simulink model "AOO_VOO_Mode"  (R2023b)
settings: Solver=VariableStepAuto  StartTime=0.0  StopTime=10.0  RelTol=1e-3
undefined symbols (not defined in the file): D10, D11, D12, D13, D2, D4, D5, D7, D8, D9, PTA0, PTA2, PTB23, PTB9, PTC3, PTC4, PTD0, PTD1, PTD2, PTD3
libraries: frdmk64flib x10
settings Model: Creator=haley  LastModifiedBy=haley

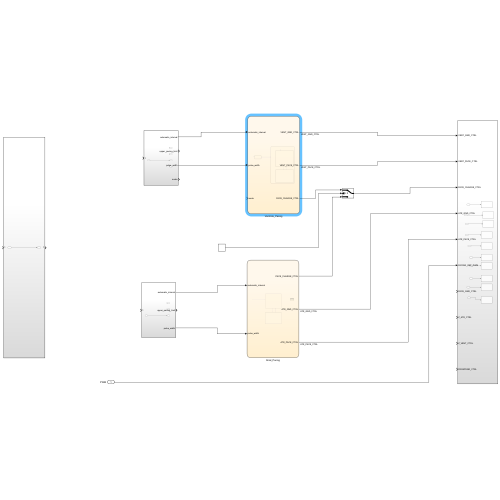
[thumbnail: Simulink's stored preview of the top-level diagram]
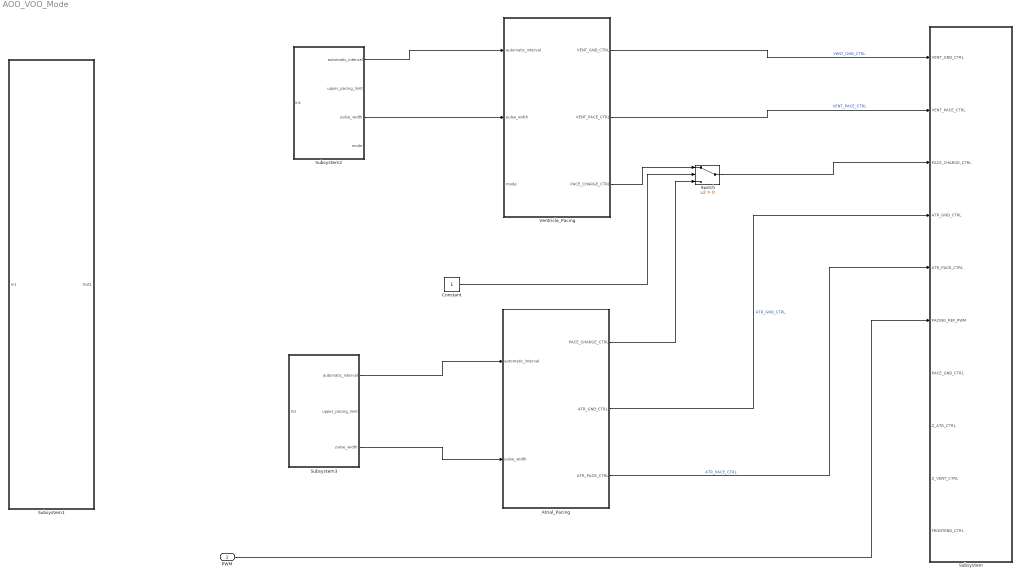
== system AOO_VOO_Mode ==
  PWM : Inport
  Atrial_Pacing : Stateflow chart  TreatAsAtomicUnit=on
      settings: PortSchema="{\"entries\":[{\"content\":{\"sides\":[{\"content\":{\"connectorIds\":[\"In1\",\"In2\"]},\"type\":\"ConnectorPlacement.EquallySpacedRectSide\",\"uuid\":\"6ace970b-fc7b-4005-8ccb-142a63debcff\"},{\"content\":{\"connectorIds\":[\"Out3\",\"Out1\",\"Out2\"],\"side\":\"RIGHT\"},\"type\":\"ConnectorPlacement.EquallySpacedRectSide\",\"uuid\":\"0deb2614-a2e1-4496-84db-77d28fbdbb57\"},{\"content\":{\"side\":\"TOP\"},\"type\":\"ConnectorPlacement.EquallySpacedRectSide\",\"uuid\":\"61e8bc8f-4916-4099-9f9f-a52b337855c5\"}]},\"type\":\"ConnectorPlacement.EquallySpacedConnector\",\"uuid\":\"8bb90a34-9390-4f4e-8609-a453406fd466\"}],\"packageUris\":[\"http://schema.mathworks.com/mf0/Connector/R2020b\"],\"version\":\"1.0\"}"
  Constant : Constant
  Subsystem : Subsystem
  Subsystem1 : Subsystem
  Subsystem2 : Subsystem
  Subsystem3 : Subsystem
  Switch : Switch  Criteria=u2 > Threshold  SaturateOnIntegerOverflow=off  InputSameDT=off
  Ventricle_Pacing : Stateflow chart  TreatAsAtomicUnit=on
      settings: PortSchema="{\"entries\":[{\"content\":{\"sides\":[{\"content\":{\"connectorIds\":[\"In1\",\"In2\",\"In3\"]},\"type\":\"ConnectorPlacement.EquallySpacedRectSide\",\"uuid\":\"0295b976-af9f-4ca7-b783-b7574ce7d878\"},{\"content\":{\"connectorIds\":[\"Out2\",\"Out3\",\"Out1\"],\"side\":\"RIGHT\"},\"type\":\"ConnectorPlacement.EquallySpacedRectSide\",\"uuid\":\"8c797538-aae3-442d-b1de-b915081191d7\"},{\"content\":{\"side\":\"TOP\"},\"type\":\"ConnectorPlacement.EquallySpacedRectSide\",\"uuid\":\"af2b1efe-c74a-43e4-9bc2-de3c8cc2477c\"}]},\"type\":\"ConnectorPlacement.EquallySpacedConnector\",\"uuid\":\"3104347d-7f4e-4d45-9d00-2e2759d20ead\"}],\"packageUris\":[\"http://schema.mathworks.com/mf0/Connector/R2020b\"],\"version\":\"1.0\"}"
  wires:
  Subsystem2/3(pulse_width) -> Ventricle_Pacing/2(pulse_width)
  Subsystem3/1(automatic_interval) -> Atrial_Pacing/1(automatic_interval)
  Atrial_Pacing/1(ATR_GND_CTRL) -> Subsystem/4(ATR_GND_CTRL)  "ATR_GND_CTRL"
  Subsystem3/3(pulse_width) -> Atrial_Pacing/2(pulse_width)
  Atrial_Pacing/2(ATR_PACE_CTRL) -> Subsystem/5(ATR_PACE_CTRL)  "ATR_PACE_CTRL"
  PWM/1 -> Subsystem/6(PACING_REF_PWM)
  Ventricle_Pacing/2(VENT_GND_CTRL) -> Subsystem/1(VENT_GND_CTRL)  "VENT_GND_CTRL"
  Ventricle_Pacing/3(VENT_PACE_CTRL) -> Subsystem/2(VENT_PACE_CTRL)  "VENT_PACE_CTRL"
  Ventricle_Pacing/1(PACE_CHARGE_CTRL) -> Switch/1
  Atrial_Pacing/3(PACE_CHARGE_CTRL) -> Switch/3
  Switch/1 -> Subsystem/3(PACE_CHARGE_CTRL)
  Constant/1 -> Switch/2
  Subsystem2/1(automatic_interval) -> Ventricle_Pacing/1(automatic_interval)

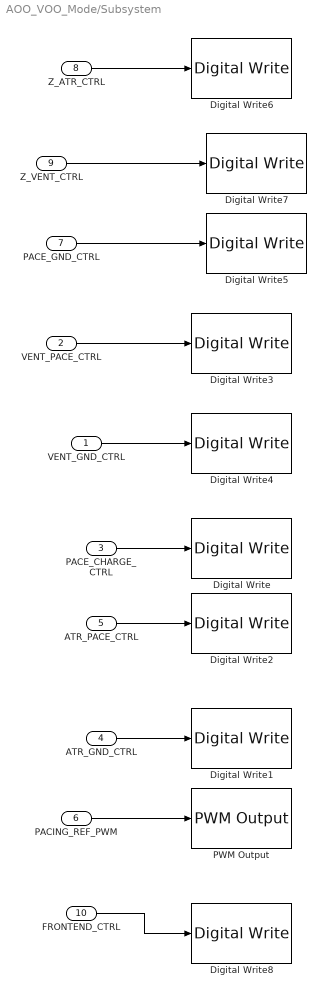
== system AOO_VOO_Mode/Subsystem ==
  VENT_GND_CTRL : Inport
  VENT_PACE_CTRL : Inport  Port=2
  PACE_CHARGE_CTRL : Inport  Port=3
  ATR_GND_CTRL : Inport  Port=4
  ATR_PACE_CTRL : Inport  Port=5
  PACING_REF_PWM : Inport  Port=6
  PACE_GND_CTRL : Inport  Port=7
  Z_ATR_CTRL : Inport  Port=8
  Z_VENT_CTRL : Inport  Port=9
  FRONTEND_CTRL : Inport  Port=10
  Digital Write : frdmk64flib/Digital Write  Whichpin=PTB9 (D2)
  Digital Write1 : frdmk64flib/Digital Write  Whichpin=PTD2 (D11)
  Digital Write2 : frdmk64flib/Digital Write  Whichpin=PTA0 (D8)
  Digital Write3 : frdmk64flib/Digital Write  Whichpin=PTC4 (D9)
  Digital Write4 : frdmk64flib/Digital Write  Whichpin=PTD3 (D12)
  Digital Write5 : frdmk64flib/Digital Write  Whichpin=PTD0 (D10)
  Digital Write6 : frdmk64flib/Digital Write  Whichpin=PTB23 (D4)
  Digital Write7 : frdmk64flib/Digital Write  Whichpin=PTC3 (D7)
  Digital Write8 : frdmk64flib/Digital Write  Whichpin=PTD1 (D13)
  PWM Output : frdmk64flib/PWM Output  Whichpin=PTA2 (D5)  InitialFrequency=2000  InitialDutyCycle=0
  wires:
  PACE_CHARGE_CTRL/1 -> Digital Write/1
  ATR_GND_CTRL/1 -> Digital Write1/1
  ATR_PACE_CTRL/1 -> Digital Write2/1
  VENT_PACE_CTRL/1 -> Digital Write3/1
  VENT_GND_CTRL/1 -> Digital Write4/1
  PACING_REF_PWM/1 -> PWM Output/1
  PACE_GND_CTRL/1 -> Digital Write5/1
  Z_ATR_CTRL/1 -> Digital Write6/1
  Z_VENT_CTRL/1 -> Digital Write7/1
  FRONTEND_CTRL/1 -> Digital Write8/1

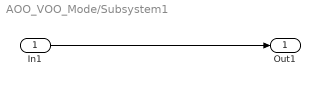
== system AOO_VOO_Mode/Subsystem1 ==
  In1 : Inport
  Out1 : Outport
  wires:
  In1/1 -> Out1/1

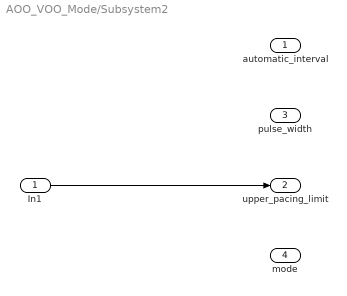
== system AOO_VOO_Mode/Subsystem2 ==
  In1 : Inport
  automatic_interval : Outport
  upper_pacing_limit : Outport  Port=2
  pulse_width : Outport  Port=3
  mode : Outport  Port=4
  wires:
  In1/1 -> upper_pacing_limit/1

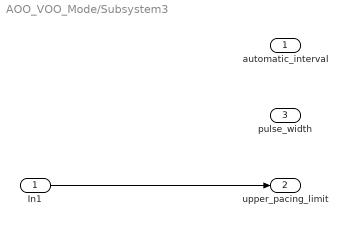
== system AOO_VOO_Mode/Subsystem3 ==
  In1 : Inport
  automatic_interval : Outport
  upper_pacing_limit : Outport  Port=2
  pulse_width : Outport  Port=3
  wires:
  In1/1 -> upper_pacing_limit/1

== stateflow chart AOO_VOO_Mode/Atrial_Pacing ==
  state Charge_C22_Discharge_C21
    entry:
    %Charge C22
    ATR_PACE_CTRL = 0;
    PACE_CHARGE_CTRL = 1;
    %Discharge C21
    ATR_GND_CTRL = 1;
  state ?
  state ChargeC21_and_DischargeC22
    %Creates the leading edge and sends pulse for X amount of time
    entry:
    PACE_CHARGE_CTRL = 0;
    ATR_PACE_CTRL = 1;
    ATR_GND_CTRL = 0;
    %Recharge pulse is the current in the opposite direction due to C21
  (default) -> Charge_C22_Discharge_C21
  Charge_C22_Discharge_C21 -> ChargeC21_and_DischargeC22 : after(automatic_interval-pulse_width, msec)
  ChargeC21_and_DischargeC22 -> Charge_C22_Discharge_C21 : after(pulse_width, msec)
  data: automatic_interval input; pulse_width input; ATR_GND_CTRL output; ATR_PACE_CTRL output; PACE_CHARGE_CTRL output

== stateflow chart AOO_VOO_Mode/Ventricle_Pacing ==
  state AOO
    state Charge_C22_Discharge_C21
      entry:
      %Charge C22
      VENT_PACE_CTRL = 0;
      PACE_CHARGE_CTRL = 1;
      %Discharge C21
      VENT_GND_CTRL= 1;
    state ChargeC21_and_DischargeC22
      %Creates the leading edge and sends pulse for X amount of time
      entry:
      PACE_CHARGE_CTRL = 0;
      VENT_GND_CTRL = 0;
      VENT_PACE_CTRL = 1;
      %Recharge pulse is the current in the opposite direction due to C21
    (default) -> Charge_C22_Discharge_C21
    Charge_C22_Discharge_C21 -> ChargeC21_and_DischargeC22 : after(automatic_interval-pulse_width, msec)
    ChargeC21_and_DischargeC22 -> Charge_C22_Discharge_C21 : after(pulse_width, msec)
  state Mode_Selection
  (default) -> Mode_Selection
  Mode_Selection -> AOO : [mode==0]
  data: automatic_interval input; pulse_width input; PACE_CHARGE_CTRL output; VENT_GND_CTRL output; VENT_PACE_CTRL output; mode input
